simulink model "sfcndemo_sfun_bitop"  (Simulink 6.0)
settings: Solver=FixedStepDiscrete  SolverMode=SingleTasking  StartTime=0.0  StopTime=10.0  RelTol=1e-3
libraries: simulink x10
settings Model: Creator=The MathWorks Inc.  LastModifiedBy=batserve  ExtModeTrigMode=oneshot  ExtModeArmWhenConnect=off  ExtModeAutoUpdateStatusClock=off
settings DataIOCC: LimitDataPoints=off
settings OptimizationCC: BlockReduction=off  BooleanDataType=off  InlineInvariantSignals=off  OptimizeModelRefInitCode=on  LifeSpan=1
settings DebuggingCC: CheckExecutionContextPreStartOutputMsg=on  CheckExecutionContextRuntimeOutputMsg=on  SolverPrmCheckMsg=none
settings RTWCC: SystemTargetFile=ert.tlc  TemplateMakefile=ert_default_tmf  Description=RTW Embedded Coder (no auto configuration)  ProcessScript=ert_make_rtw_hook
settings CodeAppCC: IgnoreCustomStorageClasses=off
settings ERTTargetCC: TargetFcnLib=ansi_tfl_tmw.mat  GenFloatMathFcnCalls=ANSI_C  GenerateSampleERTMain=on  MatFileLogging=on  SupportContinuousTime=on  SupportNonInlinedSFcns=on  RootIOFormat=Individual Arguments  ERTCustomFileTemplate=example_file_process.tlc  InitialValueSource=Model

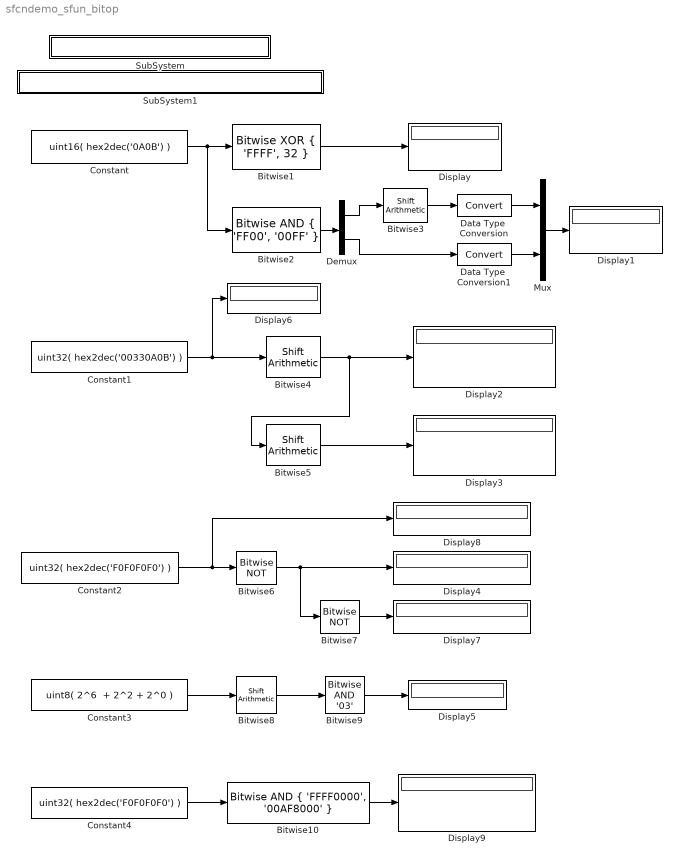
== system sfcndemo_sfun_bitop ==
  Bitwise1 : simulink/Logic and Bit Operations/Bitwise Operator  logicop=XOR  UseBitMask=on  BitMask={ 'FFFF', 32 }  BitMaskRealWorld=Stored Integer
  Bitwise10 : simulink/Logic and Bit Operations/Bitwise Operator  logicop=AND  UseBitMask=on  BitMask={ 'FFFF0000', '00AF8000' }  BitMaskRealWorld=Stored Integer
  Bitwise2 : simulink/Logic and Bit Operations/Bitwise Operator  logicop=AND  UseBitMask=on  BitMask={ 'FF00', '00FF' }  BitMaskRealWorld=Stored Integer
  Bitwise3 : simulink/Logic and Bit Operations/Shift Arithmetic  nBitShiftRight=8  nBinPtShiftRight=0
  Bitwise4 : simulink/Logic and Bit Operations/Shift Arithmetic  nBitShiftRight=-([ 1, 2, 3 ])  nBinPtShiftRight=0
  Bitwise5 : simulink/Logic and Bit Operations/Shift Arithmetic  nBitShiftRight=[ 1, 2, 3 ]  nBinPtShiftRight=0
  Bitwise6 : simulink/Logic and Bit Operations/Bitwise Operator  logicop=NOT  UseBitMask=on  BitMask=1  BitMaskRealWorld=Stored Integer
  Bitwise7 : simulink/Logic and Bit Operations/Bitwise Operator  logicop=NOT  UseBitMask=on  BitMask=1  BitMaskRealWorld=Stored Integer
  Bitwise8 : simulink/Logic and Bit Operations/Shift Arithmetic  nBitShiftRight=5  nBinPtShiftRight=0
  Bitwise9 : simulink/Logic and Bit Operations/Bitwise Operator  logicop=AND  UseBitMask=on  BitMask='03'  BitMaskRealWorld=Stored Integer
  Constant : Constant  Value=uint16( hex2dec('0A0B') )
  Constant1 : Constant  Value=uint32( hex2dec('00330A0B') )
  Constant2 : Constant  Value=uint32( hex2dec('F0F0F0F0') )
  Constant3 : Constant  Value="uint8( 2^6  + 2^2 + 2^0 )"
  Constant4 : Constant  Value=uint32( hex2dec('F0F0F0F0') )
  Data Type  Conversion : DataTypeConversion  OutDataTypeMode=uint8  SaturateOnIntegerOverflow=on  RndMeth=Zero
  Data Type  Conversion1 : DataTypeConversion  OutDataTypeMode=uint8  SaturateOnIntegerOverflow=on  RndMeth=Zero
  Demux : Demux  Outputs=2
  Display{,1..9} (10 alike) : Display
  Mux : Mux  Inputs=2
  SubSystem : Subsystem  PropExecContextAcrossSSBoundary=on
      settings: OpenFcn=edit(fullfile(matlabroot,'simulink','src','sfun_bitop.c'))
      mask Display: disp('matlabroot\simulink\src\sfun_bitop.c');
  SubSystem1 : Subsystem  PropExecContextAcrossSSBoundary=on
      settings: OpenFcn=edit(fullfile(matlabroot,'toolbox','simulink','blocks','tlc_c','sfun_bitop.tlc'))
      mask Display: disp('matlabroot\toolbox\simulink\blocks\tlc_c\sfun_bitop.tlc');
  wires:
  Constant/1 -> Bitwise1/1, Bitwise2/1
  Bitwise1/1 -> Display/1
  Bitwise4/1 -> Bitwise5/1, Display2/1
  Bitwise5/1 -> Display3/1
  Constant1/1 -> Bitwise4/1, Display6/1
  Constant3/1 -> Bitwise8/1
  Bitwise8/1 -> Bitwise9/1
  Bitwise9/1 -> Display5/1
  Constant2/1 -> Bitwise6/1, Display8/1
  Bitwise6/1 -> Display4/1, Bitwise7/1
  Bitwise7/1 -> Display7/1
  Constant4/1 -> Bitwise10/1
  Bitwise10/1 -> Display9/1
  Bitwise2/1 -> Demux/1
  Demux/1 -> Bitwise3/1
  Bitwise3/1 -> Data Type  Conversion/1
  Data Type  Conversion/1 -> Mux/1
  Mux/1 -> Display1/1
  Demux/2 -> Data Type  Conversion1/1
  Data Type  Conversion1/1 -> Mux/2

== system sfcndemo_sfun_bitop/SubSystem ==

== system sfcndemo_sfun_bitop/SubSystem1 ==
